simulink model "3K04_Assignment1"  (R2021b)
settings: Solver=FixedStepAuto  StartTime=0.0  StopTime=1  FixedStep=1e-3  RelTol=1e-3  EnableMultiTasking=on
undefined symbols (not defined in the file): D0, D1, D10, D11, D12, D13, D2, D3, D4, D5, D6, D7, D8, D9, PTA0, PTA1, PTA2, PTB23, PTB9, PTC16, PTC17, PTC2, PTC3, PTC4, PTD0, PTD1, PTD2, PTD3
libraries: frdmk64flib x14
settings Model: ExtModeTrigDuration=5  Creator=Stephen Oh  LastModifiedBy=Mian Chen
settings SolverCC: AlgebraicLoopSolver=TrustRegion
settings OptimizationCC: EnhancedBackFolding=on  PassReuseOutputArgsAs=Individual arguments  ZeroExternalMemoryAtStartup=off  ZeroInternalMemoryAtStartup=off  MaxStackSize=64  OptimizeBlockOrder=speed  DifferentSizesBufferReuse=on  OptimizationCustomize=off  EfficientTunableParamExpr=on
settings DebuggingCC: ParameterTunabilityLossMsg=error  SFMachineParentedDataDiag=warning
settings HardwareCC: ProdBitPerPointer=32  ProdBitPerSizeT=32  ProdBitPerPtrDiffT=32  ProdLargestAtomicInteger=Long  ProdLargestAtomicFloat=Double  ProdWordSize=32  ProdHWDeviceType=ARM Compatible->ARM Cortex  UseEmbeddedCoderFeatures=off
settings SFSimCC: MATLABDynamicMemAlloc=off
settings RTWCC: Description=Embedded Coder  SystemTargetFile=ert.tlc  HardwareBoard=NXP FRDM-K64F  TLCOptions="-aInlineSetEventsForThisBaseRateFcn=TLC_FALSE -aSuppressMultiTaskScheduler=TLC_FALSE  -aRateBasedStepFcn=0"  TemplateMakefile=ert_default_tmf  Toolchain=GNU Tools for ARM Embedded Processors
settings CodeAppCC: ForceParamTrailComments=on  IgnoreCustomStorageClasses=off  OperatorAnnotations=on  SimulinkDataObjDesc=on  SFDataObjDesc=on  InsertBlockDesc=on
settings ERTTargetCC: SupportNonInlinedSFcns=on

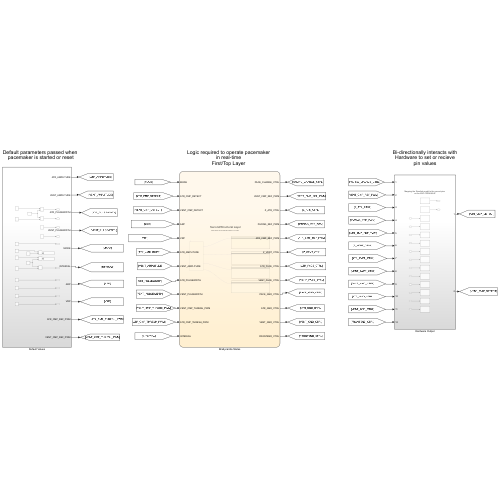
[thumbnail: Simulink's stored preview of the top-level diagram]
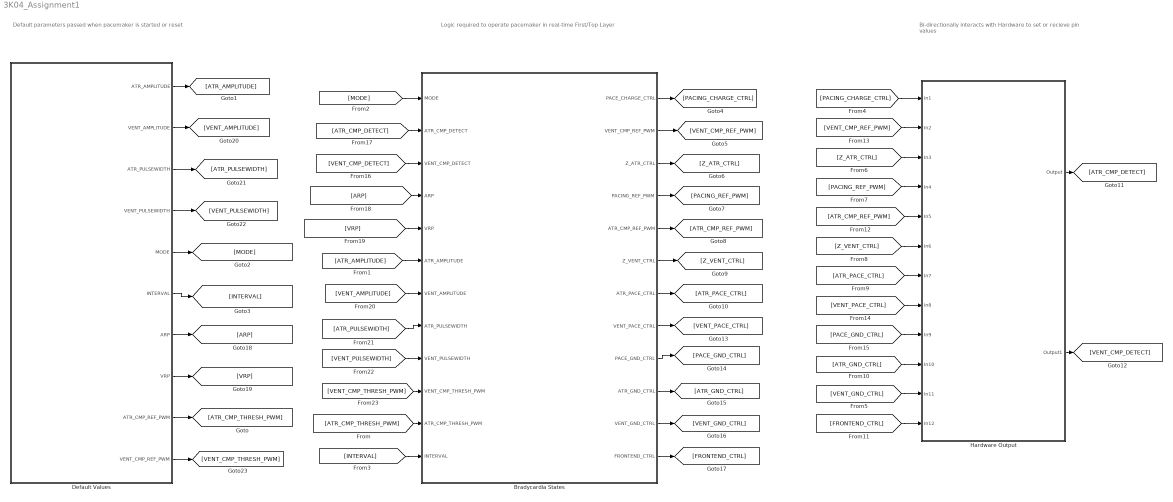
== system 3K04_Assignment1 ==
  note: Default parameters passed when
      | pacemaker is started or reset
  note: Logic required to operate pacemaker
      | in real-time
      | First/Top Layer
  note: Bi-directionally interacts with
      | Hardware to set or recieve
      | pin values
  Bradycardia States : Stateflow chart  TreatAsAtomicUnit=on
      settings: PortSchema="{\"entries\":[{\"content\":{\"sides\":[{\"content\":{\"connectorIds\":[\"In2\",\"In3\",\"In4\",\"In5\",\"In6\",\"In7\",\"In8\",\"In9\",\"In10\",\"In11\",\"In12\",\"In1\"]},\"type\":\"ConnectorPlacement.EquallySpacedRectSide\",\"uuid\":\"15e03f69-5c25-4f3e-b3fb-d71978e552f4\"},{\"content\":{\"connectorIds\":[\"Out7\",\"Out12\",\"Out4\",\"Out8\",\"Out10\",\"Out5\",\"Out9\",\"Out3\",\"Out6\",\"Out1\",\"Out2\",\"Out11\"],\"side\":\"RIGHT\"},\"type\":\"ConnectorPlacement.EquallySpacedRectSide\",\"uuid\":\"02171bf1-edb1-4b01-9e56-a8642c556ed6\"},{\"content\":{\"connectorIds\":[],\"side\":\"TOP\"},\"type\":\"ConnectorPlacement.EquallySpacedRectSide\",\"uuid\":\"cc6b5506-3435-4740-9e3f-4dfe15d30bff\"}]},\"type\":\"ConnectorPlacement.EquallySpacedConnector\",\"uuid\":\"0ad55da7-1e65-48d0-a0a4-2620ffa94320\"}],\"packageUris\":[\"http://schema.mathworks.com/mf0/Connector/19700101\"],\"version\":\"1.0\"}"
  Default Values : Subsystem
  Hardware Output : Subsystem
  wires:
  [INTERVAL] -> Bradycardia States/1(INTERVAL)
  [ATR_GND_CTRL] -> Hardware Output/10(In10)
  [PACING_REF_PWM] -> Hardware Output/4(In4)
  [Z_VENT_CTRL] -> Hardware Output/6(In6)
  [ATR_PACE_CTRL] -> Hardware Output/7(In7)
  Hardware Output/2(Output1) -> [VENT_CMP_DETECT]
  [PACE_GND_CTRL] -> Hardware Output/9(In9)
  [FRONTEND_CTRL] -> Hardware Output/12(In12)
  [VENT_GND_CTRL] -> Hardware Output/11(In11)
  [Z_ATR_CTRL] -> Hardware Output/3(In3)
  [VENT_PACE_CTRL] -> Hardware Output/8(In8)
  [ATR_CMP_REF_PWM] -> Hardware Output/5(In5)
  [VENT_CMP_REF_PWM] -> Hardware Output/2(In2)
  [PACING_CHARGE_CTRL] -> Hardware Output/1(In1)
  Hardware Output/1(Output) -> [ATR_CMP_DETECT]
  [MODE] -> Bradycardia States/2(MODE)
  [ARP] -> Bradycardia States/5(ARP)
  [VRP] -> Bradycardia States/6(VRP)
  [ATR_CMP_DETECT] -> Bradycardia States/3(ATR_CMP_DETECT)
  [ATR_AMPLITUDE] -> Bradycardia States/7(ATR_AMPLITUDE)
  [VENT_AMPLITUDE] -> Bradycardia States/8(VENT_AMPLITUDE)
  [ATR_PULSEWIDTH] -> Bradycardia States/9(ATR_PULSEWIDTH)
  [VENT_PULSEWIDTH] -> Bradycardia States/10(VENT_PULSEWIDTH)
  Default Values/2(VENT_AMPLITUDE) -> [VENT_AMPLITUDE]
  Default Values/8(VRP) -> [VRP]
  Default Values/5(MODE) -> [MODE]
  Default Values/4(VENT_PULSEWIDTH) -> [VENT_PULSEWIDTH]
  Default Values/3(ATR_PULSEWIDTH) -> [ATR_PULSEWIDTH]
  Default Values/1(ATR_AMPLITUDE) -> [ATR_AMPLITUDE]
  Default Values/6(INTERVAL) -> [INTERVAL]
  Default Values/7(ARP) -> [ARP]
  Bradycardia States/3(VENT_PACE_CTRL) -> [VENT_PACE_CTRL]
  Bradycardia States/9(ATR_PACE_CTRL) -> [ATR_PACE_CTRL]
  Bradycardia States/7(PACE_CHARGE_CTRL) -> [PACING_CHARGE_CTRL]
  Bradycardia States/12(VENT_CMP_REF_PWM) -> [VENT_CMP_REF_PWM]
  Bradycardia States/4(Z_ATR_CTRL) -> [Z_ATR_CTRL]
  Bradycardia States/8(PACING_REF_PWM) -> [PACING_REF_PWM]
  Bradycardia States/10(ATR_CMP_REF_PWM) -> [ATR_CMP_REF_PWM]
  Bradycardia States/5(Z_VENT_CTRL) -> [Z_VENT_CTRL]
  Bradycardia States/6(PACE_GND_CTRL) -> [PACE_GND_CTRL]
  Bradycardia States/1(ATR_GND_CTRL) -> [ATR_GND_CTRL]
  Bradycardia States/2(VENT_GND_CTRL) -> [VENT_GND_CTRL]
  Bradycardia States/11(FRONTEND_CTRL) -> [FRONTEND_CTRL]
  Default Values/10(VENT_CMP_REF_PWM) -> [VENT_CMP_THRESH_PWM]
  Default Values/9(ATR_CMP_REF_PWM) -> [ATR_CMP_THRESH_PWM]
  [ATR_CMP_THRESH_PWM] -> Bradycardia States/12(ATR_CMP_THRESH_PWM)
  [VENT_CMP_THRESH_PWM] -> Bradycardia States/11(VENT_CMP_THRESH_PWM)
  [VENT_CMP_DETECT] -> Bradycardia States/4(VENT_CMP_DETECT)

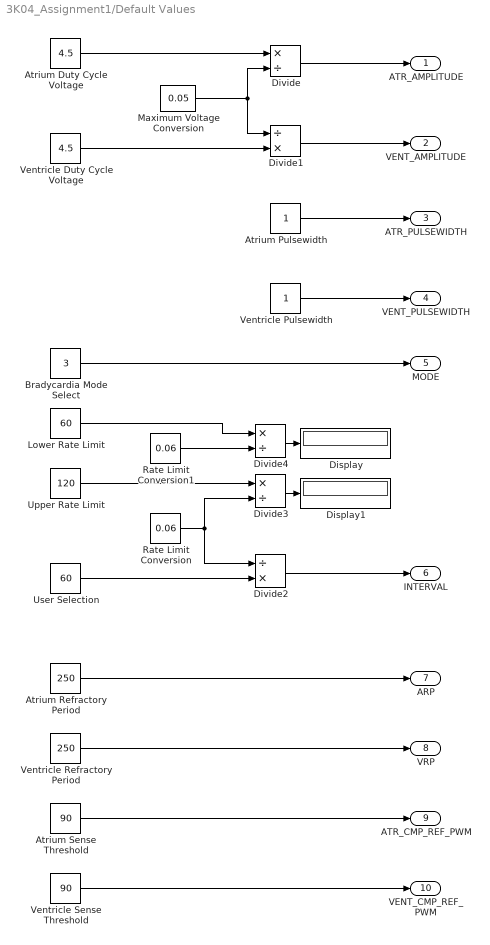
== system 3K04_Assignment1/Default Values ==
  Atrium Duty Cycle Voltage : Constant  Value=4.5
  Atrium Pulsewidth : Constant
  Atrium Refractory Period : Constant  Value=250
  Atrium Sense Threshold : Constant  Value=90
  Bradycardia Mode Select : Constant  Value=3
  Display : Display
  Display1 : Display
  Divide : Product  Inputs=*/
  Divide1 : Product  Inputs=/*
  Divide2 : Product  Inputs=/*
  Divide3 : Product  Inputs=*/
  Divide4 : Product  Inputs=*/
  Lower Rate Limit : Constant  Value=60
  Maximum Voltage Conversion : Constant  Value=0.05
  Rate Limit Conversion : Constant  Value=0.06
  Rate Limit Conversion1 : Constant  Value=0.06
  Upper Rate Limit : Constant  Value=120
  User Selection : Constant  Value=60
  Ventricle Duty Cycle Voltage : Constant  Value=4.5
  Ventricle Pulsewidth : Constant
  Ventricle Refractory Period : Constant  Value=250
  Ventricle Sense Threshold : Constant  Value=90
  ATR_AMPLITUDE : Outport
  VENT_AMPLITUDE : Outport  Port=2
  ATR_PULSEWIDTH : Outport  Port=3
  VENT_PULSEWIDTH : Outport  Port=4
  MODE : Outport  Port=5
  INTERVAL : Outport  Port=6
  ARP : Outport  Port=7
  VRP : Outport  Port=8
  ATR_CMP_REF_PWM : Outport  Port=9
  VENT_CMP_REF_PWM : Outport  Port=10
  wires:
  Atrium Duty Cycle Voltage/1 -> Divide/1
  Ventricle Pulsewidth/1 -> VENT_PULSEWIDTH/1
  Bradycardia Mode Select/1 -> MODE/1
  Divide2/1 -> INTERVAL/1
  Atrium Refractory Period/1 -> ARP/1
  Ventricle Refractory Period/1 -> VRP/1
  Atrium Pulsewidth/1 -> ATR_PULSEWIDTH/1
  Atrium Sense Threshold/1 -> ATR_CMP_REF_PWM/1
  Ventricle Sense Threshold/1 -> VENT_CMP_REF_PWM/1
  Maximum Voltage Conversion/1 -> Divide1/1, Divide/2
  Divide/1 -> ATR_AMPLITUDE/1
  Divide1/1 -> VENT_AMPLITUDE/1
  Ventricle Duty Cycle Voltage/1 -> Divide1/2
  User Selection/1 -> Divide2/2
  Rate Limit Conversion/1 -> Divide3/2, Divide2/1
  Upper Rate Limit/1 -> Divide3/1
  Lower Rate Limit/1 -> Divide4/1
  Rate Limit Conversion1/1 -> Divide4/2
  Divide4/1 -> Display/1
  Divide3/1 -> Display1/1

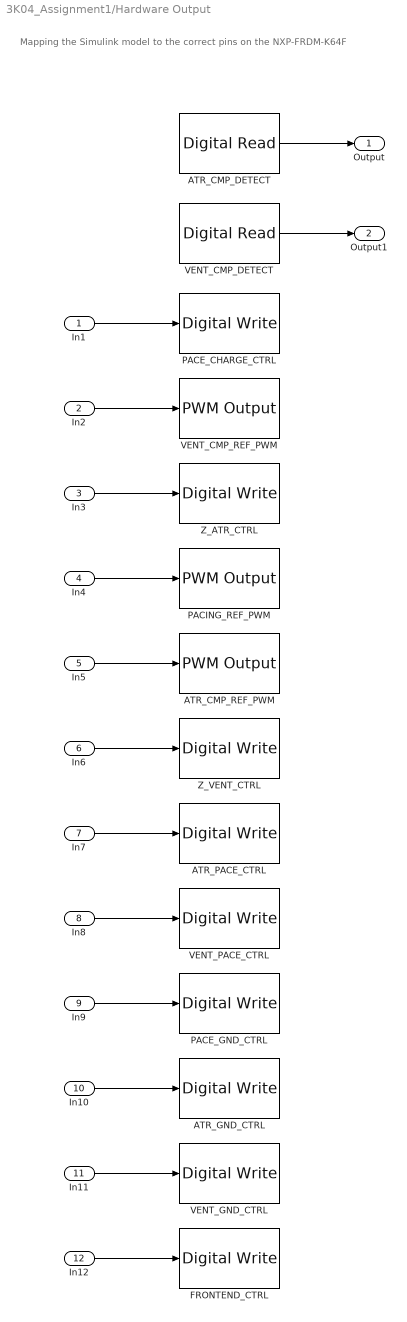
== system 3K04_Assignment1/Hardware Output ==
  note: Mapping the Simulink model to the correct pins
      | on the NXP-FRDM-K64F
  In1 : Inport
  In2 : Inport  Port=2
  In3 : Inport  Port=3
  In4 : Inport  Port=4
  In5 : Inport  Port=5
  In6 : Inport  Port=6
  In7 : Inport  Port=7
  In8 : Inport  Port=8
  In9 : Inport  Port=9
  In10 : Inport  Port=10
  In11 : Inport  Port=11
  In12 : Inport  Port=12
  ATR_CMP_DETECT : frdmk64flib/Digital Read  Whichpin=PTC16 (D0)  SampleTime=-1
  ATR_CMP_REF_PWM : frdmk64flib/PWM Output  Whichpin=PTC2 (D6)  InitialFrequency=2000  InitialDutyCycle=30
  ATR_GND_CTRL : frdmk64flib/Digital Write  Whichpin=PTD2 (D11)
  ATR_PACE_CTRL : frdmk64flib/Digital Write  Whichpin=PTA0 (D8)
  FRONTEND_CTRL : frdmk64flib/Digital Write  Whichpin=PTD1 (D13)
  PACE_CHARGE_CTRL : frdmk64flib/Digital Write  Whichpin=PTB9 (D2)
  PACE_GND_CTRL : frdmk64flib/Digital Write  Whichpin=PTD0 (D10)
  PACING_REF_PWM : frdmk64flib/PWM Output  Whichpin=PTA2 (D5)  InitialFrequency=2000  InitialDutyCycle=30
  VENT_CMP_DETECT : frdmk64flib/Digital Read  Whichpin=PTC17 (D1)  SampleTime=-1
  VENT_CMP_REF_PWM : frdmk64flib/PWM Output  Whichpin=PTA1 (D3)  InitialFrequency=2000  InitialDutyCycle=30
  VENT_GND_CTRL : frdmk64flib/Digital Write  Whichpin=PTD3 (D12)
  VENT_PACE_CTRL : frdmk64flib/Digital Write  Whichpin=PTC4 (D9)
  Z_ATR_CTRL : frdmk64flib/Digital Write  Whichpin=PTB23 (D4)
  Z_VENT_CTRL : frdmk64flib/Digital Write  Whichpin=PTC3 (D7)
  Output : Outport
  Output1 : Outport  Port=2
  wires:
  In1/1 -> PACE_CHARGE_CTRL/1
  ATR_CMP_DETECT/1 -> Output/1
  VENT_CMP_DETECT/1 -> Output1/1
  In2/1 -> VENT_CMP_REF_PWM/1
  In3/1 -> Z_ATR_CTRL/1
  In4/1 -> PACING_REF_PWM/1
  In5/1 -> ATR_CMP_REF_PWM/1
  In6/1 -> Z_VENT_CTRL/1
  In7/1 -> ATR_PACE_CTRL/1
  In8/1 -> VENT_PACE_CTRL/1
  In9/1 -> PACE_GND_CTRL/1
  In10/1 -> ATR_GND_CTRL/1
  In11/1 -> VENT_GND_CTRL/1
  In12/1 -> FRONTEND_CTRL/1

== stateflow chart 3K04_Assignment1/Bradycardia States ==
  note: Second/Structural Layer
  note: Mode Select with Conditional transition to 4 modes
  state AOO [group]
    state Charging
      entry:
      %
      %Charging capacitor C22
      %
      ATR_PACE_CTRL = LOW
      VENT_PACE_CTRL = LOW
      PACING_REF_PWM = ATR_AMPLITUDE
      PACE_CHARGE_CTRL = HIGH
      %
      %Charge release of capacitor C21 into Atrium ground
      %
      PACE_GND_CTRL = HIGH
      VENT_PACE_CTRL = LOW
      Z_ATR_CTRL = LOW
      Z_VENT_CTRL = LOW
      ATR_PACE_CTRL = LOW
      ATR_GND_CTRL = HIGH
      VENT_GND_CTRL = LOW
    state Discharging
      entry:
      %
      %Charge release of capacitor C22 to charge capacitor C21
      %
      PACE_CHARGE_CTRL = LOW
      PACE_GND_CTRL = HIGH
      VENT_PACE_CTRL = LOW
      VENT_GND_CTRL = LOW
      Z_VENT_CTRL = LOW
      Z_ATR_CTRL = LOW
      ATR_GND_CTRL = LOW
      ATR_PACE_CTRL = HIGH
    AOO.Charging -> AOO.Discharging : after(INTERVAL, msec)
    AOO.Discharging -> AOO.Charging : after(ATR_PULSEWIDTH, msec)
  state ModeSelect
  state VOO [group]
    state Charging
      entry:
      %
      %Charging capacitor C22
      %
      ATR_PACE_CTRL = LOW
      VENT_PACE_CTRL = LOW
      PACING_REF_PWM = VENT_AMPLITUDE
      PACE_CHARGE_CTRL = HIGH
      %
      %Charge release of capacitor C21 into Ventricle ground
      %
      PACE_GND_CTRL = HIGH
      VENT_PACE_CTRL = LOW
      Z_ATR_CTRL = LOW
      Z_VENT_CTRL = LOW
      ATR_PACE_CTRL = LOW
      ATR_GND_CTRL = LOW
      VENT_GND_CTRL = HIGH
    state Discharging
      entry:
      %
      %Charge release of capacitor C22 to charge capacitor C21
      %
      PACE_CHARGE_CTRL = LOW
      PACE_GND_CTRL = HIGH
      ATR_PACE_CTRL = LOW
      ATR_GND_CTRL = LOW
      Z_VENT_CTRL = LOW
      Z_ATR_CTRL = LOW
      VENT_GND_CTRL = LOW
      VENT_PACE_CTRL = HIGH
    VOO.Charging -> VOO.Discharging : after(INTERVAL, msec)
    VOO.Discharging -> VOO.Charging : after(VENT_PULSEWIDTH, msec)
  state AAI [group]
    state Transition
      %Check for sense outside atrium refractory period
    state Discharging
      entry:
      %Charge release of capacitor C22 to charge capacitor C21
      %
      PACE_CHARGE_CTRL = LOW
      PACE_GND_CTRL = HIGH
      VENT_PACE_CTRL = LOW
      VENT_GND_CTRL = LOW
      Z_VENT_CTRL = LOW
      Z_ATR_CTRL = LOW
      ATR_GND_CTRL = LOW
      ATR_PACE_CTRL = HIGH
    state Charging
      entry:
      %
      %Turn sensing on
      FRONTEND_CTRL = HIGH
      ATR_CMP_REF_PWM = ATR_CMP_THRESH_PWM
      %Charging capacitor C22
      %
      ATR_PACE_CTRL = LOW
      VENT_PACE_CTRL = LOW
      PACING_REF_PWM = ATR_AMPLITUDE
      PACE_CHARGE_CTRL = HIGH
      %Charge release of capacitor C21 into Atrium ground
      PACE_GND_CTRL = HIGH
      VENT_PACE_CTRL = LOW
      Z_ATR_CTRL = LOW
      Z_VENT_CTRL = LOW
      ATR_PACE_CTRL = LOW
      ATR_GND_CTRL = HIGH
      VENT_GND_CTRL = LOW
    AAI.Transition -> AAI.Charging [order 2] : [ATR_CMP_DETECT == HIGH]
    AAI.Transition -> AAI.Discharging [order 1] : after(INTERVAL-ARP, msec)
    AAI.Charging -> AAI.Transition : after(ARP, msec)
    AAI.Discharging -> AAI.Charging : after(ATR_PULSEWIDTH, msec)
  state VVI [group]
    state Transition
      %Check for sense outside ventricle refractory period
    state Charging
      entry:
      %
      %Turn sensing on
      FRONTEND_CTRL = HIGH
      VENT_CMP_REF_PWM = VENT_CMP_THRESH_PWM
      %Charging capacitor C22
      %
      ATR_PACE_CTRL = LOW
      VENT_PACE_CTRL = LOW
      PACING_REF_PWM = VENT_AMPLITUDE
      PACE_CHARGE_CTRL = HIGH
      %Charge release of capacitor C21 into Ventricle ground
      PACE_GND_CTRL = HIGH
      VENT_PACE_CTRL = LOW
      Z_ATR_CTRL = LOW
      Z_VENT_CTRL = LOW
      ATR_PACE_CTRL = LOW
      ATR_GND_CTRL = LOW
      VENT_GND_CTRL = HIGH
    state Discharging
      entry:
      %Charge release of capacitor C22 to charge capacitor C21
      %
      PACE_CHARGE_CTRL = LOW
      PACE_GND_CTRL = HIGH
      ATR_PACE_CTRL = LOW
      ATR_GND_CTRL = LOW
      Z_VENT_CTRL = LOW
      Z_ATR_CTRL = LOW
      VENT_GND_CTRL = LOW
      VENT_PACE_CTRL = HIGH
    VVI.Transition -> VVI.Discharging [order 1] : after(INTERVAL-VRP, msec)
    VVI.Transition -> VVI.Charging [order 2] : [VENT_CMP_DETECT == HIGH]
    VVI.Charging -> VVI.Transition : after(VRP, msec)
    VVI.Discharging -> VVI.Charging : after(VENT_PULSEWIDTH, msec)
  (default) -> ModeSelect
  ModeSelect -> AOO.Charging [order 1] : [MODE == 0]
  ModeSelect -> VOO.Charging [order 2] : [MODE == 1]
  ModeSelect -> VVI.Charging [order 4] : [MODE == 3]
  ModeSelect -> AAI.Charging [order 3] : [MODE == 2]
  data: ATR_GND_CTRL output; VENT_GND_CTRL output; VENT_PACE_CTRL output; Z_ATR_CTRL output; Z_VENT_CTRL output; PACE_GND_CTRL output; PACE_CHARGE_CTRL output; PACING_REF_PWM output; ATR_PACE_CTRL output; INTERVAL input; HIGH local boolean =true; LOW local boolean =false; MODE input; ATR_CMP_REF_PWM output; FRONTEND_CTRL output; VENT_CMP_REF_PWM output; ATR_CMP_DETECT input; VENT_CMP_DETECT input; ARP input; VRP input; ATR_AMPLITUDE input; VENT_AMPLITUDE input; ATR_PULSEWIDTH input; VENT_PULSEWIDTH input; VENT_CMP_THRESH_PWM input; ATR_CMP_THRESH_PWM input
